simulink model "RLFactoryEnforceCrash6Opponents"  (R2020a)
settings: Solver=VariableStepAuto  StartTime=0.0  StopTime=60  RelTol=1e-3
undefined symbols (not defined in the file): BLOCKEDTIMER, EPS, getRandomSafeCoord, GoalRange, MAXVELOA, MAXVELOB, MAXVELOC, MAXVELOD, MAXVELOE, MAXVELOF, rl, RLStartX, RLStartY, SAFETYDISTANCEA, SAFETYDISTANCEB, SAFETYDISTANCEC, SAFETYDISTANCED, SAFETYDISTANCEE, SAFETYDISTANCEF, THRESHOLDA, THRESHOLDB, THRESHOLDC, THRESHOLDD, THRESHOLDE, THRESHOLDF, TSA, TSB, TSC, TSD, TSE, TSF, TSRL
libraries: rllib x1
(part 3 of 3)

== system RLFactoryEnforceCrash6Opponents/RLServiceDOpponent/RLServiceAOpponentController/RLServiceInvalidMoveChecker ==
  MoveX : Inport
  MoveY : Inport  Port=2
  DiffRLX : Inport  Port=3
  DiffRLY : Inport  Port=4
  THRESHOLD : Inport  Port=5
  Constant5 : Constant
  Constant6 : Constant  Value=0
  Constant7 : Constant  Value=0
  Constant8 : Constant
  Constant9 : Constant
  Product : Product
  Product1 : Product
  Square : Math  Operator=square  SaturateOnIntegerOverflow=on
  Square Root : Sqrt  SaturateOnIntegerOverflow=on
  Square1 : Math  Operator=square  SaturateOnIntegerOverflow=on
  Sum : Sum  Inputs=+|-
  Sum1 : Sum
  Sum5 : Sum  Inputs=+|+
  Sum6 : Sum  Inputs=+|-|+
  Switch1 : Switch  Criteria=u2 > Threshold
  Switch3 : Switch  Criteria=u2 > Threshold
  MoveInValid : Outport
  wires:
  Product1/1 -> Sum5/2
  Sum5/1 -> Switch3/2
  Product/1 -> Sum5/1
  Sum6/1 -> MoveInValid/1
  Switch3/1 -> Sum6/1
  Constant9/1 -> Switch3/1
  MoveY/1 -> Product1/1
  MoveX/1 -> Product/1
  Constant8/1 -> Sum6/2
  Constant7/1 -> Switch3/3
  THRESHOLD/1 -> Sum/2
  Sum/1 -> Switch1/2
  Constant5/1 -> Switch1/3
  Constant6/1 -> Switch1/1
  Switch1/1 -> Sum6/3
  DiffRLY/1 -> Square1/1, Product1/2
  DiffRLX/1 -> Product/2, Square/1
  Square1/1 -> Sum1/2
  Sum1/1 -> Square Root/1
  Square/1 -> Sum1/1
  Square Root/1 -> Sum/1

== system RLFactoryEnforceCrash6Opponents/RLServiceDOpponent/RLServiceAOpponentController/RLServicePMAdjustVelocity ==
  MoveX : Inport
  MoveY : Inport  Port=2
  Velocity : Inport  Port=3
  Constant : Constant
  Demux1 : Demux  Outputs=2
  Divide : Product  Inputs=*/
  Divide1 : Product  Inputs=*/
  Mux : Mux  Inputs=2
  Product : Product
  Product3 : Product
  Sqrt1 : Sqrt  SaturateOnIntegerOverflow=on
  Square : Math  Operator=square  SaturateOnIntegerOverflow=on
  Square1 : Math  Operator=square  SaturateOnIntegerOverflow=on
  Sum : Sum  Inputs=+|+
  Switch : Switch  Criteria=u2 > Threshold
  AdjX : Outport
  AdjY : Outport  Port=2
  wires:
  Velocity/1 -> Product/2, Product3/2
  MoveX/1 -> Square/1, Mux/1
  MoveY/1 -> Square1/1, Mux/2
  Divide1/1 -> Product3/1
  Divide/1 -> Product/1
  Switch/1 -> Divide1/2, Divide/2
  Constant/1 -> Switch/3
  Mux/1 -> Demux1/1
  Demux1/2 -> Divide1/1
  Square1/1 -> Sum/2
  Sum/1 -> Sqrt1/1
  Demux1/1 -> Divide/1
  Product/1 -> AdjX/1
  Sqrt1/1 -> Switch/2, Switch/1
  Product3/1 -> AdjY/1
  Square/1 -> Sum/1

== system RLFactoryEnforceCrash6Opponents/RLServiceDOpponent/RLServiceAOpponentController/RLServiceXAvoidOvershooting ==
  MoveX : Inport
  MoveY : Inport  Port=2
  DiffToGoalX : Inport  Port=3
  DiffToGoalY : Inport  Port=4
  TS : Inport  Port=5
  Abs{1..4} (4 alike) : Abs
  Divide : Product  Inputs=*/
  Divide1 : Product  Inputs=*/
  Product : Product
  Product1 : Product
  Sum1 : Sum  Inputs=-|+
  Sum2 : Sum  Inputs=-|+
  Switch : Switch  Criteria=u2 > Threshold
  Switch1 : Switch  Criteria=u2 > Threshold
  MoveXNoOvershoot : Outport
  MoveYNoOvershoot : Outport  Port=2
  wires:
  Abs1/1 -> Sum1/2
  Switch/1 -> MoveXNoOvershoot/1
  Product/1 -> Abs2/1
  Abs2/1 -> Sum1/1
  DiffToGoalX/1 -> Divide/1, Abs1/1
  Sum1/1 -> Switch/2
  MoveX/1 -> Product/1, Switch/1
  Divide/1 -> Switch/3
  MoveY/1 -> Product1/1, Switch1/1
  Sum2/1 -> Switch1/2
  Abs4/1 -> Sum2/1
  Product1/1 -> Abs4/1
  Divide1/1 -> Switch1/3
  TS/1 -> Divide1/2, Product1/2, Divide/2, Product/2
  Abs3/1 -> Sum2/2
  Switch1/1 -> MoveYNoOvershoot/1
  DiffToGoalY/1 -> Divide1/1, Abs3/1

== system RLFactoryEnforceCrash6Opponents/RLServiceEOpponent/RLServiceAOpponentController/RLServiceArrivedChecker ==
  X : Inport
  Y : Inport  Port=2
  GoalX : Inport  Port=3
  GoalY : Inport  Port=4
  RLX : Inport  Port=5
  RLY : Inport  Port=6
  THRESHOLD : Inport  Port=7
  Constant1 : Constant
  Constant3 : Constant
  Constant4 : Constant  Value=0
  Constant5 : Constant  Value=0
  Constant6 : Constant
  Constant8 : Constant  Value=-BLOCKEDTIMER
  Integrator : Integrator  LimitOutput=on  UpperSaturationLimit=BLOCKEDTIMER  LowerSaturationLimit=0
  RLServiceEuclideanDistanceCalculator1 : Subsystem
  RLServiceEuclideanDistanceCalculator2 : Subsystem
  Sum : Sum  Inputs=|++
  Sum1 : Sum  Inputs=+-|
  Switch1 : Switch  Criteria=u2 > Threshold  Threshold=0.5
  Switch3 : Switch  Threshold=BLOCKEDTIMER
  Switch4 : Switch  Criteria=u2 > Threshold
  ArrivedCheck : Outport
  wires:
  RLServiceEuclideanDistanceCalculator1/1(DistToGoal) -> Switch1/2
  X/1 -> RLServiceEuclideanDistanceCalculator1/1(X)
  Switch1/1 -> Sum/1
  Constant3/1 -> Switch1/3
  Y/1 -> RLServiceEuclideanDistanceCalculator1/2(Y)
  Constant4/1 -> Switch1/1
  Sum/1 -> ArrivedCheck/1
  Switch3/1 -> Sum/2
  Integrator/1 -> Switch3/2
  Constant5/1 -> Switch3/3
  RLX/1 -> RLServiceEuclideanDistanceCalculator2/1(X)
  RLY/1 -> RLServiceEuclideanDistanceCalculator2/2(Y)
  GoalX/1 -> RLServiceEuclideanDistanceCalculator2/3(GoalX), RLServiceEuclideanDistanceCalculator1/3(GoalX)
  GoalY/1 -> RLServiceEuclideanDistanceCalculator2/4(GoalY), RLServiceEuclideanDistanceCalculator1/4(GoalY)
  RLServiceEuclideanDistanceCalculator2/1(OppDistToGoal) -> Sum1/1
  Constant8/1 -> Switch4/1
  Constant6/1 -> Switch4/3
  THRESHOLD/1 -> Sum1/2
  Sum1/1 -> Switch4/2
  Switch4/1 -> Integrator/1
  Constant1/1 -> Switch3/1

== system RLFactoryEnforceCrash6Opponents/RLServiceEOpponent/RLServiceAOpponentController/RLServiceEMAdjustVelocity ==
  MoveX : Inport
  MoveY : Inport  Port=2
  Velocity : Inport  Port=3
  Constant : Constant
  Demux1 : Demux  Outputs=2
  Divide : Product  Inputs=*/
  Divide1 : Product  Inputs=*/
  Mux : Mux  Inputs=2
  Product : Product
  Product3 : Product
  Sqrt1 : Sqrt  SaturateOnIntegerOverflow=on
  Square : Math  Operator=square  SaturateOnIntegerOverflow=on
  Square1 : Math  Operator=square  SaturateOnIntegerOverflow=on
  Sum : Sum  Inputs=+|+
  Switch : Switch  Criteria=u2 > Threshold
  AdjX : Outport
  AdjY : Outport  Port=2
  wires:
  Product/1 -> AdjX/1
  MoveY/1 -> Square1/1, Mux/2
  Mux/1 -> Demux1/1
  Divide1/1 -> Product3/1
  Constant/1 -> Switch/3
  Square1/1 -> Sum/2
  Switch/1 -> Divide1/2, Divide/2
  Velocity/1 -> Product/2, Product3/2
  Sum/1 -> Sqrt1/1
  Square/1 -> Sum/1
  Sqrt1/1 -> Switch/2, Switch/1
  Product3/1 -> AdjY/1
  Demux1/2 -> Divide1/1
  MoveX/1 -> Square/1, Mux/1
  Demux1/1 -> Divide/1
  Divide/1 -> Product/1

== system RLFactoryEnforceCrash6Opponents/RLServiceEOpponent/RLServiceAOpponentController/RLServiceEvasiveMoveChooser ==
  DiffRLX : Inport
  DiffRLY : Inport  Port=2
  DiffGoalX : Inport  Port=3
  DiffGoalY : Inport  Port=4
  Abs : Abs
  Abs1 : Abs
  Demux{,2..4} (4 alike) : Demux  Outputs=2
  Gain : Gain  Gain=-1
  Gain1 : Gain  Gain=-1
  Mux1 : Mux  Inputs=2
  Mux2 : Mux  Inputs=2
  Mux3 : Mux  Inputs=2
  Sqrt : Sqrt  SaturateOnIntegerOverflow=on
  Sqrt1 : Sqrt  SaturateOnIntegerOverflow=on
  Sum{,1..2,5} (4 alike) : Sum  Inputs=+|+
  Sum6 : Sum  Inputs=+|-
  Switch : Switch  Criteria=u2 > Threshold
  Switch1 : Switch  Criteria=u2 > Threshold
  EMX : Outport
  EMY : Outport  Port=2
  wires:
  Gain/1 -> Mux1/1
  DiffRLX/1 -> Gain1/1, Mux1/2
  Gain1/1 -> Mux2/2
  DiffGoalX/1 -> Mux3/1
  DiffGoalY/1 -> Mux3/2
  Mux3/1 -> Sum/2, Sum1/2
  Mux2/1 -> Sum/1, Demux4/1
  Mux1/1 -> Demux3/1, Sum1/1
  Sum1/1 -> Abs/1
  Sum/1 -> Abs1/1
  Abs1/1 -> Demux/1
  Demux/1 -> Sum2/1
  Demux/2 -> Sum2/2
  Demux2/2 -> Sum5/2
  Demux2/1 -> Sum5/1
  Abs/1 -> Demux2/1
  Sum5/1 -> Sqrt/1
  Sum2/1 -> Sqrt1/1
  Sqrt/1 -> Sum6/1
  Sqrt1/1 -> Sum6/2
  Sum6/1 -> Switch/2, Switch1/2
  Demux3/1 -> Switch/1
  Demux3/2 -> Switch1/1
  Demux4/1 -> Switch/3
  Demux4/2 -> Switch1/3
  Switch/1 -> EMX/1
  Switch1/1 -> EMY/1
  DiffRLY/1 -> Mux2/1, Gain/1

== system RLFactoryEnforceCrash6Opponents/RLServiceEOpponent/RLServiceAOpponentController/RLServiceInvalidMoveChecker ==
  MoveX : Inport
  MoveY : Inport  Port=2
  DiffRLX : Inport  Port=3
  DiffRLY : Inport  Port=4
  THRESHOLD : Inport  Port=5
  Constant5 : Constant
  Constant6 : Constant  Value=0
  Constant7 : Constant  Value=0
  Constant8 : Constant
  Constant9 : Constant
  Product : Product
  Product1 : Product
  Square : Math  Operator=square  SaturateOnIntegerOverflow=on
  Square Root : Sqrt  SaturateOnIntegerOverflow=on
  Square1 : Math  Operator=square  SaturateOnIntegerOverflow=on
  Sum : Sum  Inputs=+|-
  Sum1 : Sum
  Sum5 : Sum  Inputs=+|+
  Sum6 : Sum  Inputs=+|-|+
  Switch1 : Switch  Criteria=u2 > Threshold
  Switch3 : Switch  Criteria=u2 > Threshold
  MoveInValid : Outport
  wires:
  Product1/1 -> Sum5/2
  Sum5/1 -> Switch3/2
  Product/1 -> Sum5/1
  Sum6/1 -> MoveInValid/1
  Switch3/1 -> Sum6/1
  Constant9/1 -> Switch3/1
  MoveY/1 -> Product1/1
  MoveX/1 -> Product/1
  Constant8/1 -> Sum6/2
  Constant7/1 -> Switch3/3
  THRESHOLD/1 -> Sum/2
  Sum/1 -> Switch1/2
  Constant5/1 -> Switch1/3
  Constant6/1 -> Switch1/1
  Switch1/1 -> Sum6/3
  DiffRLY/1 -> Square1/1, Product1/2
  DiffRLX/1 -> Product/2, Square/1
  Square1/1 -> Sum1/2
  Sum1/1 -> Square Root/1
  Square/1 -> Sum1/1
  Square Root/1 -> Sum/1

== system RLFactoryEnforceCrash6Opponents/RLServiceEOpponent/RLServiceAOpponentController/RLServicePMAdjustVelocity ==
  MoveX : Inport
  MoveY : Inport  Port=2
  Velocity : Inport  Port=3
  Constant : Constant
  Demux1 : Demux  Outputs=2
  Divide : Product  Inputs=*/
  Divide1 : Product  Inputs=*/
  Mux : Mux  Inputs=2
  Product : Product
  Product3 : Product
  Sqrt1 : Sqrt  SaturateOnIntegerOverflow=on
  Square : Math  Operator=square  SaturateOnIntegerOverflow=on
  Square1 : Math  Operator=square  SaturateOnIntegerOverflow=on
  Sum : Sum  Inputs=+|+
  Switch : Switch  Criteria=u2 > Threshold
  AdjX : Outport
  AdjY : Outport  Port=2
  wires:
  Velocity/1 -> Product/2, Product3/2
  MoveX/1 -> Square/1, Mux/1
  MoveY/1 -> Square1/1, Mux/2
  Divide1/1 -> Product3/1
  Divide/1 -> Product/1
  Switch/1 -> Divide1/2, Divide/2
  Constant/1 -> Switch/3
  Mux/1 -> Demux1/1
  Demux1/2 -> Divide1/1
  Square1/1 -> Sum/2
  Sum/1 -> Sqrt1/1
  Demux1/1 -> Divide/1
  Product/1 -> AdjX/1
  Sqrt1/1 -> Switch/2, Switch/1
  Product3/1 -> AdjY/1
  Square/1 -> Sum/1

== system RLFactoryEnforceCrash6Opponents/RLServiceEOpponent/RLServiceAOpponentController/RLServiceXAvoidOvershooting ==
  MoveX : Inport
  MoveY : Inport  Port=2
  DiffToGoalX : Inport  Port=3
  DiffToGoalY : Inport  Port=4
  TS : Inport  Port=5
  Abs{1..4} (4 alike) : Abs
  Divide : Product  Inputs=*/
  Divide1 : Product  Inputs=*/
  Product : Product
  Product1 : Product
  Sum1 : Sum  Inputs=-|+
  Sum2 : Sum  Inputs=-|+
  Switch : Switch  Criteria=u2 > Threshold
  Switch1 : Switch  Criteria=u2 > Threshold
  MoveXNoOvershoot : Outport
  MoveYNoOvershoot : Outport  Port=2
  wires:
  Abs1/1 -> Sum1/2
  Switch/1 -> MoveXNoOvershoot/1
  Product/1 -> Abs2/1
  Abs2/1 -> Sum1/1
  DiffToGoalX/1 -> Divide/1, Abs1/1
  Sum1/1 -> Switch/2
  MoveX/1 -> Product/1, Switch/1
  Divide/1 -> Switch/3
  MoveY/1 -> Product1/1, Switch1/1
  Sum2/1 -> Switch1/2
  Abs4/1 -> Sum2/1
  Product1/1 -> Abs4/1
  Divide1/1 -> Switch1/3
  TS/1 -> Divide1/2, Product1/2, Divide/2, Product/2
  Abs3/1 -> Sum2/2
  Switch1/1 -> MoveYNoOvershoot/1
  DiffToGoalY/1 -> Divide1/1, Abs3/1

== system RLFactoryEnforceCrash6Opponents/RLServiceFOpponent/RLServiceAOpponentController/RLServiceArrivedChecker ==
  X : Inport
  Y : Inport  Port=2
  GoalX : Inport  Port=3
  GoalY : Inport  Port=4
  RLX : Inport  Port=5
  RLY : Inport  Port=6
  THRESHOLD : Inport  Port=7
  Constant1 : Constant
  Constant3 : Constant
  Constant4 : Constant  Value=0
  Constant5 : Constant  Value=0
  Constant6 : Constant
  Constant8 : Constant  Value=-BLOCKEDTIMER
  Integrator : Integrator  LimitOutput=on  UpperSaturationLimit=BLOCKEDTIMER  LowerSaturationLimit=0
  RLServiceEuclideanDistanceCalculator1 : Subsystem
  RLServiceEuclideanDistanceCalculator2 : Subsystem
  Sum : Sum  Inputs=|++
  Sum1 : Sum  Inputs=+-|
  Switch1 : Switch  Criteria=u2 > Threshold  Threshold=0.5
  Switch3 : Switch  Threshold=BLOCKEDTIMER
  Switch4 : Switch  Criteria=u2 > Threshold
  ArrivedCheck : Outport
  wires:
  RLServiceEuclideanDistanceCalculator1/1(DistToGoal) -> Switch1/2
  X/1 -> RLServiceEuclideanDistanceCalculator1/1(X)
  Switch1/1 -> Sum/1
  Constant3/1 -> Switch1/3
  Y/1 -> RLServiceEuclideanDistanceCalculator1/2(Y)
  Constant4/1 -> Switch1/1
  Sum/1 -> ArrivedCheck/1
  Switch3/1 -> Sum/2
  Integrator/1 -> Switch3/2
  Constant5/1 -> Switch3/3
  RLX/1 -> RLServiceEuclideanDistanceCalculator2/1(X)
  RLY/1 -> RLServiceEuclideanDistanceCalculator2/2(Y)
  GoalX/1 -> RLServiceEuclideanDistanceCalculator2/3(GoalX), RLServiceEuclideanDistanceCalculator1/3(GoalX)
  GoalY/1 -> RLServiceEuclideanDistanceCalculator2/4(GoalY), RLServiceEuclideanDistanceCalculator1/4(GoalY)
  RLServiceEuclideanDistanceCalculator2/1(OppDistToGoal) -> Sum1/1
  Constant8/1 -> Switch4/1
  Constant6/1 -> Switch4/3
  THRESHOLD/1 -> Sum1/2
  Sum1/1 -> Switch4/2
  Switch4/1 -> Integrator/1
  Constant1/1 -> Switch3/1

== system RLFactoryEnforceCrash6Opponents/RLServiceFOpponent/RLServiceAOpponentController/RLServiceEMAdjustVelocity ==
  MoveX : Inport
  MoveY : Inport  Port=2
  Velocity : Inport  Port=3
  Constant : Constant
  Demux1 : Demux  Outputs=2
  Divide : Product  Inputs=*/
  Divide1 : Product  Inputs=*/
  Mux : Mux  Inputs=2
  Product : Product
  Product3 : Product
  Sqrt1 : Sqrt  SaturateOnIntegerOverflow=on
  Square : Math  Operator=square  SaturateOnIntegerOverflow=on
  Square1 : Math  Operator=square  SaturateOnIntegerOverflow=on
  Sum : Sum  Inputs=+|+
  Switch : Switch  Criteria=u2 > Threshold
  AdjX : Outport
  AdjY : Outport  Port=2
  wires:
  Product/1 -> AdjX/1
  MoveY/1 -> Square1/1, Mux/2
  Mux/1 -> Demux1/1
  Divide1/1 -> Product3/1
  Constant/1 -> Switch/3
  Square1/1 -> Sum/2
  Switch/1 -> Divide1/2, Divide/2
  Velocity/1 -> Product/2, Product3/2
  Sum/1 -> Sqrt1/1
  Square/1 -> Sum/1
  Sqrt1/1 -> Switch/2, Switch/1
  Product3/1 -> AdjY/1
  Demux1/2 -> Divide1/1
  MoveX/1 -> Square/1, Mux/1
  Demux1/1 -> Divide/1
  Divide/1 -> Product/1

== system RLFactoryEnforceCrash6Opponents/RLServiceFOpponent/RLServiceAOpponentController/RLServiceEvasiveMoveChooser ==
  DiffRLX : Inport
  DiffRLY : Inport  Port=2
  DiffGoalX : Inport  Port=3
  DiffGoalY : Inport  Port=4
  Abs : Abs
  Abs1 : Abs
  Demux{,2..4} (4 alike) : Demux  Outputs=2
  Gain : Gain  Gain=-1
  Gain1 : Gain  Gain=-1
  Mux1 : Mux  Inputs=2
  Mux2 : Mux  Inputs=2
  Mux3 : Mux  Inputs=2
  Sqrt : Sqrt  SaturateOnIntegerOverflow=on
  Sqrt1 : Sqrt  SaturateOnIntegerOverflow=on
  Sum{,1..2,5} (4 alike) : Sum  Inputs=+|+
  Sum6 : Sum  Inputs=+|-
  Switch : Switch  Criteria=u2 > Threshold
  Switch1 : Switch  Criteria=u2 > Threshold
  EMX : Outport
  EMY : Outport  Port=2
  wires:
  Gain/1 -> Mux1/1
  DiffRLX/1 -> Gain1/1, Mux1/2
  Gain1/1 -> Mux2/2
  DiffGoalX/1 -> Mux3/1
  DiffGoalY/1 -> Mux3/2
  Mux3/1 -> Sum/2, Sum1/2
  Mux2/1 -> Sum/1, Demux4/1
  Mux1/1 -> Demux3/1, Sum1/1
  Sum1/1 -> Abs/1
  Sum/1 -> Abs1/1
  Abs1/1 -> Demux/1
  Demux/1 -> Sum2/1
  Demux/2 -> Sum2/2
  Demux2/2 -> Sum5/2
  Demux2/1 -> Sum5/1
  Abs/1 -> Demux2/1
  Sum5/1 -> Sqrt/1
  Sum2/1 -> Sqrt1/1
  Sqrt/1 -> Sum6/1
  Sqrt1/1 -> Sum6/2
  Sum6/1 -> Switch/2, Switch1/2
  Demux3/1 -> Switch/1
  Demux3/2 -> Switch1/1
  Demux4/1 -> Switch/3
  Demux4/2 -> Switch1/3
  Switch/1 -> EMX/1
  Switch1/1 -> EMY/1
  DiffRLY/1 -> Mux2/1, Gain/1

== system RLFactoryEnforceCrash6Opponents/RLServiceFOpponent/RLServiceAOpponentController/RLServiceInvalidMoveChecker ==
  MoveX : Inport
  MoveY : Inport  Port=2
  DiffRLX : Inport  Port=3
  DiffRLY : Inport  Port=4
  THRESHOLD : Inport  Port=5
  Constant5 : Constant
  Constant6 : Constant  Value=0
  Constant7 : Constant  Value=0
  Constant8 : Constant
  Constant9 : Constant
  Product : Product
  Product1 : Product
  Square : Math  Operator=square  SaturateOnIntegerOverflow=on
  Square Root : Sqrt  SaturateOnIntegerOverflow=on
  Square1 : Math  Operator=square  SaturateOnIntegerOverflow=on
  Sum : Sum  Inputs=+|-
  Sum1 : Sum
  Sum5 : Sum  Inputs=+|+
  Sum6 : Sum  Inputs=+|-|+
  Switch1 : Switch  Criteria=u2 > Threshold
  Switch3 : Switch  Criteria=u2 > Threshold
  MoveInValid : Outport
  wires:
  Product1/1 -> Sum5/2
  Sum5/1 -> Switch3/2
  Product/1 -> Sum5/1
  Sum6/1 -> MoveInValid/1
  Switch3/1 -> Sum6/1
  Constant9/1 -> Switch3/1
  MoveY/1 -> Product1/1
  MoveX/1 -> Product/1
  Constant8/1 -> Sum6/2
  Constant7/1 -> Switch3/3
  THRESHOLD/1 -> Sum/2
  Sum/1 -> Switch1/2
  Constant5/1 -> Switch1/3
  Constant6/1 -> Switch1/1
  Switch1/1 -> Sum6/3
  DiffRLY/1 -> Square1/1, Product1/2
  DiffRLX/1 -> Product/2, Square/1
  Square1/1 -> Sum1/2
  Sum1/1 -> Square Root/1
  Square/1 -> Sum1/1
  Square Root/1 -> Sum/1

== system RLFactoryEnforceCrash6Opponents/RLServiceFOpponent/RLServiceAOpponentController/RLServicePMAdjustVelocity ==
  MoveX : Inport
  MoveY : Inport  Port=2
  Velocity : Inport  Port=3
  Constant : Constant
  Demux1 : Demux  Outputs=2
  Divide : Product  Inputs=*/
  Divide1 : Product  Inputs=*/
  Mux : Mux  Inputs=2
  Product : Product
  Product3 : Product
  Sqrt1 : Sqrt  SaturateOnIntegerOverflow=on
  Square : Math  Operator=square  SaturateOnIntegerOverflow=on
  Square1 : Math  Operator=square  SaturateOnIntegerOverflow=on
  Sum : Sum  Inputs=+|+
  Switch : Switch  Criteria=u2 > Threshold
  AdjX : Outport
  AdjY : Outport  Port=2
  wires:
  Velocity/1 -> Product/2, Product3/2
  MoveX/1 -> Square/1, Mux/1
  MoveY/1 -> Square1/1, Mux/2
  Divide1/1 -> Product3/1
  Divide/1 -> Product/1
  Switch/1 -> Divide1/2, Divide/2
  Constant/1 -> Switch/3
  Mux/1 -> Demux1/1
  Demux1/2 -> Divide1/1
  Square1/1 -> Sum/2
  Sum/1 -> Sqrt1/1
  Demux1/1 -> Divide/1
  Product/1 -> AdjX/1
  Sqrt1/1 -> Switch/2, Switch/1
  Product3/1 -> AdjY/1
  Square/1 -> Sum/1

== system RLFactoryEnforceCrash6Opponents/RLServiceFOpponent/RLServiceAOpponentController/RLServiceXAvoidOvershooting ==
  MoveX : Inport
  MoveY : Inport  Port=2
  DiffToGoalX : Inport  Port=3
  DiffToGoalY : Inport  Port=4
  TS : Inport  Port=5
  Abs{1..4} (4 alike) : Abs
  Divide : Product  Inputs=*/
  Divide1 : Product  Inputs=*/
  Product : Product
  Product1 : Product
  Sum1 : Sum  Inputs=-|+
  Sum2 : Sum  Inputs=-|+
  Switch : Switch  Criteria=u2 > Threshold
  Switch1 : Switch  Criteria=u2 > Threshold
  MoveXNoOvershoot : Outport
  MoveYNoOvershoot : Outport  Port=2
  wires:
  Abs1/1 -> Sum1/2
  Switch/1 -> MoveXNoOvershoot/1
  Product/1 -> Abs2/1
  Abs2/1 -> Sum1/1
  DiffToGoalX/1 -> Divide/1, Abs1/1
  Sum1/1 -> Switch/2
  MoveX/1 -> Product/1, Switch/1
  Divide/1 -> Switch/3
  MoveY/1 -> Product1/1, Switch1/1
  Sum2/1 -> Switch1/2
  Abs4/1 -> Sum2/1
  Product1/1 -> Abs4/1
  Divide1/1 -> Switch1/3
  TS/1 -> Divide1/2, Product1/2, Divide/2, Product/2
  Abs3/1 -> Sum2/2
  Switch1/1 -> MoveYNoOvershoot/1
  DiffToGoalY/1 -> Divide1/1, Abs3/1

== system RLFactoryEnforceCrash6Opponents/RLService6RLRobot/RLService6RLRobotSensor/RLServiceARobotSensorSubsystem/RLServiceDirectionCalculator ==
  OppX : Inport
  OppY : Inport  Port=2
  Demux : Demux  Outputs=2
  Mux : Mux  Inputs=2
  Sign : Signum
  Sign1 : Signum
  Sum : Sum  Inputs=+-
  Unit Delay : UnitDelay  SampleTime=TSRL  HasFrameUpgradeWarning=on
  DirOppX : Outport
  DirOppY : Outport  Port=2
  wires:
  Mux/1 -> Unit Delay/1, Sum/1
  Unit Delay/1 -> Sum/2
  Sum/1 -> Demux/1
  Demux/1 -> Sign1/1
  Demux/2 -> Sign/1
  Sign1/1 -> DirOppX/1
  Sign/1 -> DirOppY/1
  OppX/1 -> Mux/1
  OppY/1 -> Mux/2

== system RLFactoryEnforceCrash6Opponents/RLService6RLRobot/RLService6RLRobotSensor/RLServiceBRobotSensorSubsystem/RLServiceDirectionCalculator ==
  OppX : Inport
  OppY : Inport  Port=2
  Demux : Demux  Outputs=2
  Mux : Mux  Inputs=2
  Sign : Signum
  Sign1 : Signum
  Sum : Sum  Inputs=+-
  Unit Delay : UnitDelay  SampleTime=TSRL  HasFrameUpgradeWarning=on
  DirOppX : Outport
  DirOppY : Outport  Port=2
  wires:
  Mux/1 -> Unit Delay/1, Sum/1
  Unit Delay/1 -> Sum/2
  Sum/1 -> Demux/1
  Demux/1 -> Sign1/1
  Demux/2 -> Sign/1
  Sign1/1 -> DirOppX/1
  Sign/1 -> DirOppY/1
  OppX/1 -> Mux/1
  OppY/1 -> Mux/2

== system RLFactoryEnforceCrash6Opponents/RLService6RLRobot/RLService6RLRobotSensor/RLServiceCRobotSensorSubsystem/RLServiceDirectionCalculator ==
  OppX : Inport
  OppY : Inport  Port=2
  Demux : Demux  Outputs=2
  Mux : Mux  Inputs=2
  Sign : Signum
  Sign1 : Signum
  Sum : Sum  Inputs=+-
  Unit Delay : UnitDelay  SampleTime=TSRL  HasFrameUpgradeWarning=on
  DirOppX : Outport
  DirOppY : Outport  Port=2
  wires:
  Mux/1 -> Unit Delay/1, Sum/1
  Unit Delay/1 -> Sum/2
  Sum/1 -> Demux/1
  Demux/1 -> Sign1/1
  Demux/2 -> Sign/1
  Sign1/1 -> DirOppX/1
  Sign/1 -> DirOppY/1
  OppX/1 -> Mux/1
  OppY/1 -> Mux/2

== system RLFactoryEnforceCrash6Opponents/RLService6RLRobot/RLService6RLRobotSensor/RLServiceDRobotSensorSubsystem/RLServiceDirectionCalculator ==
  OppX : Inport
  OppY : Inport  Port=2
  Demux : Demux  Outputs=2
  Mux : Mux  Inputs=2
  Sign : Signum
  Sign1 : Signum
  Sum : Sum  Inputs=+-
  Unit Delay : UnitDelay  SampleTime=TSRL  HasFrameUpgradeWarning=on
  DirOppX : Outport
  DirOppY : Outport  Port=2
  wires:
  Mux/1 -> Unit Delay/1, Sum/1
  Unit Delay/1 -> Sum/2
  Sum/1 -> Demux/1
  Demux/1 -> Sign1/1
  Demux/2 -> Sign/1
  Sign1/1 -> DirOppX/1
  Sign/1 -> DirOppY/1
  OppX/1 -> Mux/1
  OppY/1 -> Mux/2

== system RLFactoryEnforceCrash6Opponents/RLService6RLRobot/RLService6RLRobotSensor/RLServiceERobotSensorSubsystem/RLServiceDirectionCalculator ==
  OppX : Inport
  OppY : Inport  Port=2
  Demux : Demux  Outputs=2
  Mux : Mux  Inputs=2
  Sign : Signum
  Sign1 : Signum
  Sum : Sum  Inputs=+-
  Unit Delay : UnitDelay  SampleTime=TSRL  HasFrameUpgradeWarning=on
  DirOppX : Outport
  DirOppY : Outport  Port=2
  wires:
  Mux/1 -> Unit Delay/1, Sum/1
  Unit Delay/1 -> Sum/2
  Sum/1 -> Demux/1
  Demux/1 -> Sign1/1
  Demux/2 -> Sign/1
  Sign1/1 -> DirOppX/1
  Sign/1 -> DirOppY/1
  OppX/1 -> Mux/1
  OppY/1 -> Mux/2

== system RLFactoryEnforceCrash6Opponents/RLService6RLRobot/RLService6RLRobotSensor/RLServiceFRobotSensorSubsystem/RLServiceDirectionCalculator ==
  OppX : Inport
  OppY : Inport  Port=2
  Demux : Demux  Outputs=2
  Mux : Mux  Inputs=2
  Sign : Signum
  Sign1 : Signum
  Sum : Sum  Inputs=+-
  Unit Delay : UnitDelay  SampleTime=TSRL  HasFrameUpgradeWarning=on
  DirOppX : Outport
  DirOppY : Outport  Port=2
  wires:
  Mux/1 -> Unit Delay/1, Sum/1
  Unit Delay/1 -> Sum/2
  Sum/1 -> Demux/1
  Demux/1 -> Sign1/1
  Demux/2 -> Sign/1
  Sign1/1 -> DirOppX/1
  Sign/1 -> DirOppY/1
  OppX/1 -> Mux/1
  OppY/1 -> Mux/2

== system RLFactoryEnforceCrash6Opponents/RLService6RLRobot/RLServiceRLInfo/RLServiceCrashDetector/RLServiceEuclideanDistanceCalculator1 ==
  X : Inport
  Y : Inport  Port=2
  XOpp : Inport  Port=3
  YOpp : Inport  Port=4
  Square : Math  Operator=square  SaturateOnIntegerOverflow=on
  Square Root : Sqrt  SaturateOnIntegerOverflow=on
  Square1 : Math  Operator=square  SaturateOnIntegerOverflow=on
  Sum1 : Sum
  Sum3 : Sum  Inputs=+-
  Sum4 : Sum  Inputs=+-
  Dist : Outport
  wires:
  XOpp/1 -> Sum3/2
  X/1 -> Sum3/1
  Sum1/1 -> Square Root/1
  Sum4/1 -> Square1/1
  Square/1 -> Sum1/1
  Y/1 -> Sum4/1
  Square Root/1 -> Dist/1
  Square1/1 -> Sum1/2
  Sum3/1 -> Square/1
  YOpp/1 -> Sum4/2

== system RLFactoryEnforceCrash6Opponents/RLService6RLRobot/RLServiceRLInfo/RLServiceCrashDetector/RLServiceEuclideanDistanceCalculator2 ==
  X : Inport
  Y : Inport  Port=2
  XOpp : Inport  Port=3
  YOpp : Inport  Port=4
  Square : Math  Operator=square  SaturateOnIntegerOverflow=on
  Square Root : Sqrt  SaturateOnIntegerOverflow=on
  Square1 : Math  Operator=square  SaturateOnIntegerOverflow=on
  Sum1 : Sum
  Sum3 : Sum  Inputs=+-
  Sum4 : Sum  Inputs=+-
  Dist : Outport
  wires:
  XOpp/1 -> Sum3/2
  X/1 -> Sum3/1
  Sum1/1 -> Square Root/1
  Sum4/1 -> Square1/1
  Square/1 -> Sum1/1
  Y/1 -> Sum4/1
  Square Root/1 -> Dist/1
  Square1/1 -> Sum1/2
  Sum3/1 -> Square/1
  YOpp/1 -> Sum4/2

== system RLFactoryEnforceCrash6Opponents/RLService6RLRobot/RLServiceRLInfo/RLServiceCrashDetector/RLServiceEuclideanDistanceCalculator3 ==
  X : Inport
  Y : Inport  Port=2
  XOpp : Inport  Port=3
  YOpp : Inport  Port=4
  Square : Math  Operator=square  SaturateOnIntegerOverflow=on
  Square Root : Sqrt  SaturateOnIntegerOverflow=on
  Square1 : Math  Operator=square  SaturateOnIntegerOverflow=on
  Sum1 : Sum
  Sum3 : Sum  Inputs=+-
  Sum4 : Sum  Inputs=+-
  Dist : Outport
  wires:
  XOpp/1 -> Sum3/2
  X/1 -> Sum3/1
  Sum1/1 -> Square Root/1
  Sum4/1 -> Square1/1
  Square/1 -> Sum1/1
  Y/1 -> Sum4/1
  Square Root/1 -> Dist/1
  Square1/1 -> Sum1/2
  Sum3/1 -> Square/1
  YOpp/1 -> Sum4/2

== system RLFactoryEnforceCrash6Opponents/RLService6RLRobot/RLServiceRLInfo/RLServiceCrashDetector/RLServiceEuclideanDistanceCalculator4 ==
  X : Inport
  Y : Inport  Port=2
  XOpp : Inport  Port=3
  YOpp : Inport  Port=4
  Square : Math  Operator=square  SaturateOnIntegerOverflow=on
  Square Root : Sqrt  SaturateOnIntegerOverflow=on
  Square1 : Math  Operator=square  SaturateOnIntegerOverflow=on
  Sum1 : Sum
  Sum3 : Sum  Inputs=+-
  Sum4 : Sum  Inputs=+-
  Dist : Outport
  wires:
  XOpp/1 -> Sum3/2
  X/1 -> Sum3/1
  Sum1/1 -> Square Root/1
  Sum4/1 -> Square1/1
  Square/1 -> Sum1/1
  Y/1 -> Sum4/1
  Square Root/1 -> Dist/1
  Square1/1 -> Sum1/2
  Sum3/1 -> Square/1
  YOpp/1 -> Sum4/2

== system RLFactoryEnforceCrash6Opponents/RLService6RLRobot/RLServiceRLInfo/RLServiceCrashDetector/RLServiceEuclideanDistanceCalculator5 ==
  X : Inport
  Y : Inport  Port=2
  XOpp : Inport  Port=3
  YOpp : Inport  Port=4
  Square : Math  Operator=square  SaturateOnIntegerOverflow=on
  Square Root : Sqrt  SaturateOnIntegerOverflow=on
  Square1 : Math  Operator=square  SaturateOnIntegerOverflow=on
  Sum1 : Sum
  Sum3 : Sum  Inputs=+-
  Sum4 : Sum  Inputs=+-
  Dist : Outport
  wires:
  XOpp/1 -> Sum3/2
  X/1 -> Sum3/1
  Sum1/1 -> Square Root/1
  Sum4/1 -> Square1/1
  Square/1 -> Sum1/1
  Y/1 -> Sum4/1
  Square Root/1 -> Dist/1
  Square1/1 -> Sum1/2
  Sum3/1 -> Square/1
  YOpp/1 -> Sum4/2

== system RLFactoryEnforceCrash6Opponents/RLService6RLRobot/RLServiceRLInfo/RLServiceCrashDetector/RLServiceEuclideanDistanceCalculator6 ==
  X : Inport
  Y : Inport  Port=2
  XOpp : Inport  Port=3
  YOpp : Inport  Port=4
  Square : Math  Operator=square  SaturateOnIntegerOverflow=on
  Square Root : Sqrt  SaturateOnIntegerOverflow=on
  Square1 : Math  Operator=square  SaturateOnIntegerOverflow=on
  Sum1 : Sum
  Sum3 : Sum  Inputs=+-
  Sum4 : Sum  Inputs=+-
  Dist : Outport
  wires:
  XOpp/1 -> Sum3/2
  X/1 -> Sum3/1
  Sum1/1 -> Square Root/1
  Sum4/1 -> Square1/1
  Square/1 -> Sum1/1
  Y/1 -> Sum4/1
  Square Root/1 -> Dist/1
  Square1/1 -> Sum1/2
  Sum3/1 -> Square/1
  YOpp/1 -> Sum4/2

== system RLFactoryEnforceCrash6Opponents/RLService6RLRobot/RLServiceRLInfo/RLServiceGoalTracker/RLServiceEuclideanDistanceCalculator ==
  X : Inport
  Y : Inport  Port=2
  GoalX : Inport  Port=3
  GoalY : Inport  Port=4
  Square : Math  Operator=square  SaturateOnIntegerOverflow=on
  Square Root : Sqrt  SaturateOnIntegerOverflow=on
  Square1 : Math  Operator=square  SaturateOnIntegerOverflow=on
  Sum1 : Sum
  Sum3 : Sum  Inputs=+-
  Sum4 : Sum  Inputs=+-
  DistGoal : Outport
  wires:
  GoalX/1 -> Sum3/2
  X/1 -> Sum3/1
  Sum1/1 -> Square Root/1
  Sum4/1 -> Square1/1
  Square/1 -> Sum1/1
  Y/1 -> Sum4/1
  Square Root/1 -> DistGoal/1
  Square1/1 -> Sum1/2
  Sum3/1 -> Square/1
  GoalY/1 -> Sum4/2

== system RLFactoryEnforceCrash6Opponents/RLServiceAOpponent/RLServiceAOpponentController/RLServiceArrivedChecker/RLServiceEuclideanDistanceCalculator1 ==
  X : Inport
  Y : Inport  Port=2
  GoalX : Inport  Port=3
  GoalY : Inport  Port=4
  Square : Math  Operator=square  SaturateOnIntegerOverflow=on
  Square Root : Sqrt  SaturateOnIntegerOverflow=on
  Square1 : Math  Operator=square  SaturateOnIntegerOverflow=on
  Sum1 : Sum
  Sum3 : Sum  Inputs=+-
  Sum4 : Sum  Inputs=+-
  DistToGoal : Outport
  wires:
  GoalX/1 -> Sum3/2
  X/1 -> Sum3/1
  Sum1/1 -> Square Root/1
  Sum4/1 -> Square1/1
  Square/1 -> Sum1/1
  Y/1 -> Sum4/1
  Square Root/1 -> DistToGoal/1
  Square1/1 -> Sum1/2
  Sum3/1 -> Square/1
  GoalY/1 -> Sum4/2

== system RLFactoryEnforceCrash6Opponents/RLServiceAOpponent/RLServiceAOpponentController/RLServiceArrivedChecker/RLServiceEuclideanDistanceCalculator2 ==
  X : Inport
  Y : Inport  Port=2
  GoalX : Inport  Port=3
  GoalY : Inport  Port=4
  Square : Math  Operator=square  SaturateOnIntegerOverflow=on
  Square Root : Sqrt  SaturateOnIntegerOverflow=on
  Square1 : Math  Operator=square  SaturateOnIntegerOverflow=on
  Sum1 : Sum
  Sum3 : Sum  Inputs=+-
  Sum4 : Sum  Inputs=+-
  OppDistToGoal : Outport
  wires:
  GoalX/1 -> Sum3/2
  X/1 -> Sum3/1
  Sum1/1 -> Square Root/1
  Sum4/1 -> Square1/1
  Square/1 -> Sum1/1
  Y/1 -> Sum4/1
  Square Root/1 -> OppDistToGoal/1
  Square1/1 -> Sum1/2
  Sum3/1 -> Square/1
  GoalY/1 -> Sum4/2

== system RLFactoryEnforceCrash6Opponents/RLServiceBOpponent/RLServiceAOpponentController/RLServiceArrivedChecker/RLServiceEuclideanDistanceCalculator1 ==
  X : Inport
  Y : Inport  Port=2
  GoalX : Inport  Port=3
  GoalY : Inport  Port=4
  Square : Math  Operator=square  SaturateOnIntegerOverflow=on
  Square Root : Sqrt  SaturateOnIntegerOverflow=on
  Square1 : Math  Operator=square  SaturateOnIntegerOverflow=on
  Sum1 : Sum
  Sum3 : Sum  Inputs=+-
  Sum4 : Sum  Inputs=+-
  DistToGoal : Outport
  wires:
  GoalX/1 -> Sum3/2
  X/1 -> Sum3/1
  Sum1/1 -> Square Root/1
  Sum4/1 -> Square1/1
  Square/1 -> Sum1/1
  Y/1 -> Sum4/1
  Square Root/1 -> DistToGoal/1
  Square1/1 -> Sum1/2
  Sum3/1 -> Square/1
  GoalY/1 -> Sum4/2

== system RLFactoryEnforceCrash6Opponents/RLServiceBOpponent/RLServiceAOpponentController/RLServiceArrivedChecker/RLServiceEuclideanDistanceCalculator2 ==
  X : Inport
  Y : Inport  Port=2
  GoalX : Inport  Port=3
  GoalY : Inport  Port=4
  Square : Math  Operator=square  SaturateOnIntegerOverflow=on
  Square Root : Sqrt  SaturateOnIntegerOverflow=on
  Square1 : Math  Operator=square  SaturateOnIntegerOverflow=on
  Sum1 : Sum
  Sum3 : Sum  Inputs=+-
  Sum4 : Sum  Inputs=+-
  OppDistToGoal : Outport
  wires:
  GoalX/1 -> Sum3/2
  X/1 -> Sum3/1
  Sum1/1 -> Square Root/1
  Sum4/1 -> Square1/1
  Square/1 -> Sum1/1
  Y/1 -> Sum4/1
  Square Root/1 -> OppDistToGoal/1
  Square1/1 -> Sum1/2
  Sum3/1 -> Square/1
  GoalY/1 -> Sum4/2

== system RLFactoryEnforceCrash6Opponents/RLServiceCOpponent/RLServiceAOpponentController/RLServiceArrivedChecker/RLServiceEuclideanDistanceCalculator1 ==
  X : Inport
  Y : Inport  Port=2
  GoalX : Inport  Port=3
  GoalY : Inport  Port=4
  Square : Math  Operator=square  SaturateOnIntegerOverflow=on
  Square Root : Sqrt  SaturateOnIntegerOverflow=on
  Square1 : Math  Operator=square  SaturateOnIntegerOverflow=on
  Sum1 : Sum
  Sum3 : Sum  Inputs=+-
  Sum4 : Sum  Inputs=+-
  DistToGoal : Outport
  wires:
  GoalX/1 -> Sum3/2
  X/1 -> Sum3/1
  Sum1/1 -> Square Root/1
  Sum4/1 -> Square1/1
  Square/1 -> Sum1/1
  Y/1 -> Sum4/1
  Square Root/1 -> DistToGoal/1
  Square1/1 -> Sum1/2
  Sum3/1 -> Square/1
  GoalY/1 -> Sum4/2

== system RLFactoryEnforceCrash6Opponents/RLServiceCOpponent/RLServiceAOpponentController/RLServiceArrivedChecker/RLServiceEuclideanDistanceCalculator2 ==
  X : Inport
  Y : Inport  Port=2
  GoalX : Inport  Port=3
  GoalY : Inport  Port=4
  Square : Math  Operator=square  SaturateOnIntegerOverflow=on
  Square Root : Sqrt  SaturateOnIntegerOverflow=on
  Square1 : Math  Operator=square  SaturateOnIntegerOverflow=on
  Sum1 : Sum
  Sum3 : Sum  Inputs=+-
  Sum4 : Sum  Inputs=+-
  OppDistToGoal : Outport
  wires:
  GoalX/1 -> Sum3/2
  X/1 -> Sum3/1
  Sum1/1 -> Square Root/1
  Sum4/1 -> Square1/1
  Square/1 -> Sum1/1
  Y/1 -> Sum4/1
  Square Root/1 -> OppDistToGoal/1
  Square1/1 -> Sum1/2
  Sum3/1 -> Square/1
  GoalY/1 -> Sum4/2

== system RLFactoryEnforceCrash6Opponents/RLServiceDOpponent/RLServiceAOpponentController/RLServiceArrivedChecker/RLServiceEuclideanDistanceCalculator1 ==
  X : Inport
  Y : Inport  Port=2
  GoalX : Inport  Port=3
  GoalY : Inport  Port=4
  Square : Math  Operator=square  SaturateOnIntegerOverflow=on
  Square Root : Sqrt  SaturateOnIntegerOverflow=on
  Square1 : Math  Operator=square  SaturateOnIntegerOverflow=on
  Sum1 : Sum
  Sum3 : Sum  Inputs=+-
  Sum4 : Sum  Inputs=+-
  DistToGoal : Outport
  wires:
  GoalX/1 -> Sum3/2
  X/1 -> Sum3/1
  Sum1/1 -> Square Root/1
  Sum4/1 -> Square1/1
  Square/1 -> Sum1/1
  Y/1 -> Sum4/1
  Square Root/1 -> DistToGoal/1
  Square1/1 -> Sum1/2
  Sum3/1 -> Square/1
  GoalY/1 -> Sum4/2

== system RLFactoryEnforceCrash6Opponents/RLServiceDOpponent/RLServiceAOpponentController/RLServiceArrivedChecker/RLServiceEuclideanDistanceCalculator2 ==
  X : Inport
  Y : Inport  Port=2
  GoalX : Inport  Port=3
  GoalY : Inport  Port=4
  Square : Math  Operator=square  SaturateOnIntegerOverflow=on
  Square Root : Sqrt  SaturateOnIntegerOverflow=on
  Square1 : Math  Operator=square  SaturateOnIntegerOverflow=on
  Sum1 : Sum
  Sum3 : Sum  Inputs=+-
  Sum4 : Sum  Inputs=+-
  OppDistToGoal : Outport
  wires:
  GoalX/1 -> Sum3/2
  X/1 -> Sum3/1
  Sum1/1 -> Square Root/1
  Sum4/1 -> Square1/1
  Square/1 -> Sum1/1
  Y/1 -> Sum4/1
  Square Root/1 -> OppDistToGoal/1
  Square1/1 -> Sum1/2
  Sum3/1 -> Square/1
  GoalY/1 -> Sum4/2

== system RLFactoryEnforceCrash6Opponents/RLServiceEOpponent/RLServiceAOpponentController/RLServiceArrivedChecker/RLServiceEuclideanDistanceCalculator1 ==
  X : Inport
  Y : Inport  Port=2
  GoalX : Inport  Port=3
  GoalY : Inport  Port=4
  Square : Math  Operator=square  SaturateOnIntegerOverflow=on
  Square Root : Sqrt  SaturateOnIntegerOverflow=on
  Square1 : Math  Operator=square  SaturateOnIntegerOverflow=on
  Sum1 : Sum
  Sum3 : Sum  Inputs=+-
  Sum4 : Sum  Inputs=+-
  DistToGoal : Outport
  wires:
  GoalX/1 -> Sum3/2
  X/1 -> Sum3/1
  Sum1/1 -> Square Root/1
  Sum4/1 -> Square1/1
  Square/1 -> Sum1/1
  Y/1 -> Sum4/1
  Square Root/1 -> DistToGoal/1
  Square1/1 -> Sum1/2
  Sum3/1 -> Square/1
  GoalY/1 -> Sum4/2

== system RLFactoryEnforceCrash6Opponents/RLServiceEOpponent/RLServiceAOpponentController/RLServiceArrivedChecker/RLServiceEuclideanDistanceCalculator2 ==
  X : Inport
  Y : Inport  Port=2
  GoalX : Inport  Port=3
  GoalY : Inport  Port=4
  Square : Math  Operator=square  SaturateOnIntegerOverflow=on
  Square Root : Sqrt  SaturateOnIntegerOverflow=on
  Square1 : Math  Operator=square  SaturateOnIntegerOverflow=on
  Sum1 : Sum
  Sum3 : Sum  Inputs=+-
  Sum4 : Sum  Inputs=+-
  OppDistToGoal : Outport
  wires:
  GoalX/1 -> Sum3/2
  X/1 -> Sum3/1
  Sum1/1 -> Square Root/1
  Sum4/1 -> Square1/1
  Square/1 -> Sum1/1
  Y/1 -> Sum4/1
  Square Root/1 -> OppDistToGoal/1
  Square1/1 -> Sum1/2
  Sum3/1 -> Square/1
  GoalY/1 -> Sum4/2

== system RLFactoryEnforceCrash6Opponents/RLServiceFOpponent/RLServiceAOpponentController/RLServiceArrivedChecker/RLServiceEuclideanDistanceCalculator1 ==
  X : Inport
  Y : Inport  Port=2
  GoalX : Inport  Port=3
  GoalY : Inport  Port=4
  Square : Math  Operator=square  SaturateOnIntegerOverflow=on
  Square Root : Sqrt  SaturateOnIntegerOverflow=on
  Square1 : Math  Operator=square  SaturateOnIntegerOverflow=on
  Sum1 : Sum
  Sum3 : Sum  Inputs=+-
  Sum4 : Sum  Inputs=+-
  DistToGoal : Outport
  wires:
  GoalX/1 -> Sum3/2
  X/1 -> Sum3/1
  Sum1/1 -> Square Root/1
  Sum4/1 -> Square1/1
  Square/1 -> Sum1/1
  Y/1 -> Sum4/1
  Square Root/1 -> DistToGoal/1
  Square1/1 -> Sum1/2
  Sum3/1 -> Square/1
  GoalY/1 -> Sum4/2

== system RLFactoryEnforceCrash6Opponents/RLServiceFOpponent/RLServiceAOpponentController/RLServiceArrivedChecker/RLServiceEuclideanDistanceCalculator2 ==
  X : Inport
  Y : Inport  Port=2
  GoalX : Inport  Port=3
  GoalY : Inport  Port=4
  Square : Math  Operator=square  SaturateOnIntegerOverflow=on
  Square Root : Sqrt  SaturateOnIntegerOverflow=on
  Square1 : Math  Operator=square  SaturateOnIntegerOverflow=on
  Sum1 : Sum
  Sum3 : Sum  Inputs=+-
  Sum4 : Sum  Inputs=+-
  OppDistToGoal : Outport
  wires:
  GoalX/1 -> Sum3/2
  X/1 -> Sum3/1
  Sum1/1 -> Square Root/1
  Sum4/1 -> Square1/1
  Square/1 -> Sum1/1
  Y/1 -> Sum4/1
  Square Root/1 -> OppDistToGoal/1
  Square1/1 -> Sum1/2
  Sum3/1 -> Square/1
  GoalY/1 -> Sum4/2
